simulink model "SF042A_HwAgSnsrls"  (R2013b)
settings: Solver=FixedStepDiscrete  SolverMode=SingleTasking  StartTime=0.0  StopTime=1  FixedStep=0.002  RelTol=1e-3
values from neighbouring files (symbols this model uses):
  ARCHGLBPRM_2MILLISEC_SEC_F32 = DataDict.Constant    [SF042A_HwAgSnsrls_DataDict.m]
  CORRDPINIONAGCON_CNT_U08 = DataDict.Constant    [SF042A_HwAgSnsrls_DataDict.m]
  FCENTROFFSCON_CNT_U08 = DataDict.Constant    [SF042A_HwAgSnsrls_DataDict.m]
  HwAgSnsrlsCorrdPinionAgHwConf = DataDict.Calibration    [SF042A_HwAgSnsrls_DataDict.m]
  HwAgSnsrlsFCentrHwConf = DataDict.Calibration    [SF042A_HwAgSnsrls_DataDict.m]
  HwAgSnsrlsSmotngCoeff = DataDict.Calibration    [SF042A_HwAgSnsrls_DataDict.m]
  HwAgSnsrlsSmotngStepThd = DataDict.Calibration    [SF042A_HwAgSnsrls_DataDict.m]
  HwAgSnsrlsStordPinionConf = DataDict.Calibration    [SF042A_HwAgSnsrls_DataDict.m]
  HwAgSnsrlsStordPinionConfThd = DataDict.Calibration    [SF042A_HwAgSnsrls_DataDict.m]
  HwAgSnsrlsVehDynDifThd = DataDict.Calibration    [SF042A_HwAgSnsrls_DataDict.m]
  HwAgSnsrlsVehDynHwConf = DataDict.Calibration    [SF042A_HwAgSnsrls_DataDict.m]
  HwAgSnsrlsVehDynMotVelThd = DataDict.Calibration    [SF042A_HwAgSnsrls_DataDict.m]
  HwAgSnsrlsVehDynPinionTqThd = DataDict.Calibration    [SF042A_HwAgSnsrls_DataDict.m]
  HwAgSnsrlsVehDynTmr1Thd = DataDict.Calibration    [SF042A_HwAgSnsrls_DataDict.m]
  HwAgSnsrlsVehDynTmr2Thd = DataDict.Calibration    [SF042A_HwAgSnsrls_DataDict.m]
  HwAgSnsrlsVehDynVehSpdThd = DataDict.Calibration    [SF042A_HwAgSnsrls_DataDict.m]
  HwAgSnsrlsVehDynYawRateThd = DataDict.Calibration    [SF042A_HwAgSnsrls_DataDict.m]
  HwAgSnsrlsWhlFrqThd = DataDict.Calibration    [SF042A_HwAgSnsrls_DataDict.m]
  HwAgSnsrlsWhlSpdHwAgCoeff1 = DataDict.Calibration    [SF042A_HwAgSnsrls_DataDict.m]
  HwAgSnsrlsWhlSpdHwAgCoeff2 = DataDict.Calibration    [SF042A_HwAgSnsrls_DataDict.m]
  HwAgSnsrlsWhlSpdHwAgThd = DataDict.Calibration    [SF042A_HwAgSnsrls_DataDict.m]
  HwAgSnsrlsWhlSpdHwConf = DataDict.Calibration    [SF042A_HwAgSnsrls_DataDict.m]
  HwAgSnsrlsWhlSpdRatThd = DataDict.Calibration    [SF042A_HwAgSnsrls_DataDict.m]
  HwAgSnsrlsWhlSpdTmrThd = DataDict.Calibration    [SF042A_HwAgSnsrls_DataDict.m]
  HwAgSnsrlsWhlSpdVehSpdThd = DataDict.Calibration    [SF042A_HwAgSnsrls_DataDict.m]
  LASTPOSNCON_CNT_U08 = DataDict.Constant    [SF042A_HwAgSnsrls_DataDict.m]
  MILLISECTO100MICROSEC_ULS_U32 = DataDict.Constant    [SF042A_HwAgSnsrls_DataDict.m]
  SysGlbPrmSysKineRat = DataDict.ImprtdCal    [SF042A_HwAgSnsrls_DataDict.m]
  SysGlbPrmSysTqRat = DataDict.ImprtdCal    [SF042A_HwAgSnsrls_DataDict.m]
  VEHDYNCON_CNT_U08 = DataDict.Constant    [SF042A_HwAgSnsrls_DataDict.m]
  WHLSPDCON_CNT_U08 = DataDict.Constant    [SF042A_HwAgSnsrls_DataDict.m]
undefined symbols (not defined in the file or in its folder): NtcNr1, SigQlfr1
libraries: NxtrAbslt x11, Fil x8, NxtrLim x4, simulink x3, NxtrNvM x1, FixdToFloat x1
(part 5 of 6)

== system SF042A_HwAgSnsrls/HwAgSnsrls/HwAgSnsrlsPer1/Arbitrator/NewHwAgConf/HwAgOffsSeln/WheelSpeed ==
  Action Port : ActionPort  ActionType=case
  CopyRight2 : Subsystem  Description=|  mask(Copyright Information){none=on}
      | Copyright info block.                                               
      |                                                                     
      | Place copyright information at the top of every subsystem in design.
      mask prompts: none "No parameters"
      mask help: Place copyright information at the top of every subsystem in design.
      mask Display:
      | NxtrConf = 'Nexteer Confidential';
      | 
      | sys = bdroot; %handle for the current model ("system")
      | first = get_param(sys,'Created');
      | if(isempty(first))
      |     first = datestr(now,'yyyy');
      | else
      |     first = first(end-3:end);  %year is last four digits
      | end
      | 
      | last = get_param(sys,'LastModifiedDate');
      | if isempty(last)
      |     last = datestr(now,'yyyy');
      | else
      |     last = last(end-3:end);
      | end
      | 
      | if strcmp(first,last)
      |     fprintf('%s -- Copyright %s Nexteer',NxtrConf,first)
      | else
      |     fprintf('%s -- %s%s- %s Nexteer',NxtrConf,char(169),first,last)
      | end
  Data Store Read1 : DataStoreRead  DataStoreName=WhlSpdHwAgOffs
  HwAgOffs : Outport
  wires:
  Data Store Read1/1 -> HwAgOffs/1

== system SF042A_HwAgSnsrls/HwAgSnsrls/HwAgSnsrlsPer1/RelHwAgCalcn/UseMotAg/GetMotAgOffs/CopyRight2 ==

== system SF042A_HwAgSnsrls/HwAgSnsrls/HwAgSnsrlsPer1/VehDynAutoCentr/LpFilOne/If Action Subsystem1/CopyRight2 ==

== system SF042A_HwAgSnsrls/HwAgSnsrls/HwAgSnsrlsPer1/VehDynAutoCentr/LpFilOne/If Action Subsystem2/CopyRight2 ==

== system SF042A_HwAgSnsrls/HwAgSnsrls/HwAgSnsrlsPer1/VehDynAutoCentr/LpFilOneEna/VehDynTmr1/CopyRight2 ==

== system SF042A_HwAgSnsrls/HwAgSnsrls/HwAgSnsrlsPer1/VehDynAutoCentr/LpFilOneEna/VehDynTmr1/GetTiSpan1 ==
  Action Port : ActionPort  ActionType=then
  CopyRight2 : Subsystem  Description=|  mask(Copyright Information){none=on}
      | Copyright info block.                                               
      |                                                                     
      | Place copyright information at the top of every subsystem in design.
      mask prompts: none "No parameters"
      mask help: Place copyright information at the top of every subsystem in design.
      mask Display:
      | NxtrConf = 'Nexteer Confidential';
      | 
      | sys = bdroot; %handle for the current model ("system")
      | first = get_param(sys,'Created');
      | if(isempty(first))
      |     first = datestr(now,'yyyy');
      | else
      |     first = first(end-3:end);  %year is last four digits
      | end
      | 
      | last = get_param(sys,'LastModifiedDate');
      | if isempty(last)
      |     last = datestr(now,'yyyy');
      | else
      |     last = last(end-3:end);
      | end
      | 
      | if strcmp(first,last)
      |     fprintf('%s -- Copyright %s Nexteer',NxtrConf,first)
      | else
      |     fprintf('%s -- %s%s- %s Nexteer',NxtrConf,char(169),first,last)
      | end
  Data Store Read : DataStoreRead  RequirementInfo={} %GIDa_74142626_ca52_4bba_8d6e_2554ddb3abed  DataStoreName=VehDynRefTmr1
  GetTiSpan100MicroSec32bit : Subsystem  RequirementInfo={} %GIDa_b1f833b8_7400_4722_b0de_2bfd26e0a16e  mask(Timer_GTS){}
      mask help: Used to get the time span between start and current time.
  Out1 : Outport
  wires:
  GetTiSpan100MicroSec32bit/1(TiSpan) -> Out1/1
  Data Store Read/1 -> GetTiSpan100MicroSec32bit/1(RefTmr)

== system SF042A_HwAgSnsrls/HwAgSnsrls/HwAgSnsrlsPer1/VehDynAutoCentr/LpFilOneEna/VehDynTmr1/If Action Subsystem3 ==
  RelHwAg : Inport
  Action Port : ActionPort  ActionType=then
  Constant1 : Constant  RequirementInfo="{'linktype_rmi_doors' '00012961 (/E-STEER Core/SubSystem Specifications/Application Functions - EA4/SF042A Handwheel Angle Sensorless)' '#SF042A_74' 'true' 'REQ:  SF042A_74' '' } %GIDa_bf3e4162_a852_43d6_8080_5a7c9c1c5760"  Value=false  OutDataTypeStr=boolean
      settings: AttributesFormatString=%<OutDataTypeStr>
  CopyRight2 : Subsystem  Description=|  mask(Copyright Information){none=on}
      | Copyright info block.                                               
      |                                                                     
      | Place copyright information at the top of every subsystem in design.
      mask prompts: none "No parameters"
      mask help: Place copyright information at the top of every subsystem in design.
      mask Display:
      | NxtrConf = 'Nexteer Confidential';
      | 
      | sys = bdroot; %handle for the current model ("system")
      | first = get_param(sys,'Created');
      | if(isempty(first))
      |     first = datestr(now,'yyyy');
      | else
      |     first = first(end-3:end);  %year is last four digits
      | end
      | 
      | last = get_param(sys,'LastModifiedDate');
      | if isempty(last)
      |     last = datestr(now,'yyyy');
      | else
      |     last = last(end-3:end);
      | end
      | 
      | if strcmp(first,last)
      |     fprintf('%s -- Copyright %s Nexteer',NxtrConf,first)
      | else
      |     fprintf('%s -- %s%s- %s Nexteer',NxtrConf,char(169),first,last)
      | end
  Data Store Write : DataStoreWrite  RequirementInfo="{'linktype_rmi_doors' '00012961 (/E-STEER Core/SubSystem Specifications/Application Functions - EA4/SF042A Handwheel Angle Sensorless)' '#SF042A_74' 'true' 'REQ:  SF042A_74' '' } %GIDa_355dd3a5_df19_4bc0_96c9_80662073f861"  DataStoreName=RelHwAgFil1  DataStoreElements=RelHwAgFil1.FilSt
  Data Store Write1 : DataStoreWrite  RequirementInfo="{'linktype_rmi_doors' '00012961 (/E-STEER Core/SubSystem Specifications/Application Functions - EA4/SF042A Handwheel Angle Sensorless)' '#SF042A_74' 'true' 'REQ:  SF042A_74' '' } %GIDa_2fc295c5_da8d_4166_ba51_0973e58fd4a2"  DataStoreName=VehDynRefTmr2
  Data Store Write2 : DataStoreWrite  RequirementInfo="{'linktype_rmi_doors' '00012961 (/E-STEER Core/SubSystem Specifications/Application Functions - EA4/SF042A Handwheel Angle Sensorless)' '#SF042A_74' 'true' 'REQ:  SF042A_74' '' } %GIDa_f80ae885_8ebf_478b_9b31_2b213f41a136"  DataStoreName=PrevVehDynFil1Ena
  GetRefTmr100MicroSec32bit : Subsystem  RequirementInfo="{'linktype_rmi_doors' '00012961 (/E-STEER Core/SubSystem Specifications/Application Functions - EA4/SF042A Handwheel Angle Sensorless)' '#SF042A_74' 'true' 'REQ:  SF042A_74' '' } %GIDa_22af453f_e23e_4d39_aa78_6aee3b18adc7"  mask(Timer_GRF){}
      mask help: Used to get the reference time in a model.
  wires:
  Constant1/1 -> Data Store Write2/1
  GetRefTmr100MicroSec32bit/1(RefTmr) -> Data Store Write1/1
  RelHwAg/1 -> Data Store Write/1

== system SF042A_HwAgSnsrls/HwAgSnsrls/HwAgSnsrlsPer1/VehDynAutoCentr/LpFilOneEna/VehDynTmr1/Set to 0 ==
  Action Port : ActionPort  ActionType=else
  Constant= : Constant  RequirementInfo={} %GIDa_d225d475_710f_4e18_8d33_cdb597cd94b8  Value=0  OutDataTypeStr=uint32
      settings: AttributesFormatString=%<OutDataTypeStr>
  CopyRight2 : Subsystem  Description=|  mask(Copyright Information){none=on}
      | Copyright info block.                                               
      |                                                                     
      | Place copyright information at the top of every subsystem in design.
      mask prompts: none "No parameters"
      mask help: Place copyright information at the top of every subsystem in design.
      mask Display:
      | NxtrConf = 'Nexteer Confidential';
      | 
      | sys = bdroot; %handle for the current model ("system")
      | first = get_param(sys,'Created');
      | if(isempty(first))
      |     first = datestr(now,'yyyy');
      | else
      |     first = first(end-3:end);  %year is last four digits
      | end
      | 
      | last = get_param(sys,'LastModifiedDate');
      | if isempty(last)
      |     last = datestr(now,'yyyy');
      | else
      |     last = last(end-3:end);
      | end
      | 
      | if strcmp(first,last)
      |     fprintf('%s -- Copyright %s Nexteer',NxtrConf,first)
      | else
      |     fprintf('%s -- %s%s- %s Nexteer',NxtrConf,char(169),first,last)
      | end
  Data Store Write1 : DataStoreWrite  RequirementInfo={} %GIDa_09f33c30_f3bd_43b6_b205_fca292d21401  DataStoreName=VehDynRefTmr1
  GetRefTmr100MicroSec32bit : Subsystem  RequirementInfo={} %GIDa_a927190b_d792_495c_8b1d_712b059613e1  mask(Timer_GRF){}
      mask help: Used to get the reference time in a model.
  Out1 : Outport
  wires:
  GetRefTmr100MicroSec32bit/1(RefTmr) -> Data Store Write1/1
  Constant=/1 -> Out1/1

== system SF042A_HwAgSnsrls/HwAgSnsrls/HwAgSnsrlsPer1/VehDynAutoCentr/LpFilTwo/If Action Subsystem3/CopyRight2 ==

== system SF042A_HwAgSnsrls/HwAgSnsrls/HwAgSnsrlsPer1/VehDynAutoCentr/LpFilTwo/If Action Subsystem4/CopyRight2 ==

== system SF042A_HwAgSnsrls/HwAgSnsrls/HwAgSnsrlsPer1/VehDynAutoCentr/LpFilTwoEna/VehDynTmr2/CopyRight2 ==

== system SF042A_HwAgSnsrls/HwAgSnsrls/HwAgSnsrlsPer1/VehDynAutoCentr/LpFilTwoEna/VehDynTmr2/GetTiSpan2 ==
  Action Port : ActionPort  ActionType=then
  CopyRight2 : Subsystem  Description=|  mask(Copyright Information){none=on}
      | Copyright info block.                                               
      |                                                                     
      | Place copyright information at the top of every subsystem in design.
      mask prompts: none "No parameters"
      mask help: Place copyright information at the top of every subsystem in design.
      mask Display:
      | NxtrConf = 'Nexteer Confidential';
      | 
      | sys = bdroot; %handle for the current model ("system")
      | first = get_param(sys,'Created');
      | if(isempty(first))
      |     first = datestr(now,'yyyy');
      | else
      |     first = first(end-3:end);  %year is last four digits
      | end
      | 
      | last = get_param(sys,'LastModifiedDate');
      | if isempty(last)
      |     last = datestr(now,'yyyy');
      | else
      |     last = last(end-3:end);
      | end
      | 
      | if strcmp(first,last)
      |     fprintf('%s -- Copyright %s Nexteer',NxtrConf,first)
      | else
      |     fprintf('%s -- %s%s- %s Nexteer',NxtrConf,char(169),first,last)
      | end
  Data Store Read : DataStoreRead  DataStoreName=VehDynRefTmr2
  GetTiSpan100MicroSec32bit : Subsystem  mask(Timer_GTS){}
      mask help: Used to get the time span between start and current time.
  Out1 : Outport
  wires:
  GetTiSpan100MicroSec32bit/1(TiSpan) -> Out1/1
  Data Store Read/1 -> GetTiSpan100MicroSec32bit/1(RefTmr)

== system SF042A_HwAgSnsrls/HwAgSnsrls/HwAgSnsrlsPer1/VehDynAutoCentr/LpFilTwoEna/VehDynTmr2/If Action Subsystem4 ==
  FildRelHwAg1 : Inport
  Action Port : ActionPort  ActionType=then
  Constant1 : Constant  Value=false  OutDataTypeStr=boolean
      settings: AttributesFormatString=%<OutDataTypeStr>
  CopyRight2 : Subsystem  Description=|  mask(Copyright Information){none=on}
      | Copyright info block.                                               
      |                                                                     
      | Place copyright information at the top of every subsystem in design.
      mask prompts: none "No parameters"
      mask help: Place copyright information at the top of every subsystem in design.
      mask Display:
      | NxtrConf = 'Nexteer Confidential';
      | 
      | sys = bdroot; %handle for the current model ("system")
      | first = get_param(sys,'Created');
      | if(isempty(first))
      |     first = datestr(now,'yyyy');
      | else
      |     first = first(end-3:end);  %year is last four digits
      | end
      | 
      | last = get_param(sys,'LastModifiedDate');
      | if isempty(last)
      |     last = datestr(now,'yyyy');
      | else
      |     last = last(end-3:end);
      | end
      | 
      | if strcmp(first,last)
      |     fprintf('%s -- Copyright %s Nexteer',NxtrConf,first)
      | else
      |     fprintf('%s -- %s%s- %s Nexteer',NxtrConf,char(169),first,last)
      | end
  Data Store Write : DataStoreWrite  DataStoreName=RelHwAgFil2  DataStoreElements=RelHwAgFil2.FilSt
  Data Store Write1 : DataStoreWrite  DataStoreName=PrevVehDynFil2Ena
  wires:
  Constant1/1 -> Data Store Write1/1
  FildRelHwAg1/1 -> Data Store Write/1

== system SF042A_HwAgSnsrls/HwAgSnsrls/HwAgSnsrlsPer1/VehDynAutoCentr/LpFilTwoEna/VehDynTmr2/Set to 0 ==
  Action Port : ActionPort  ActionType=else
  Constant= : Constant  Value=0  OutDataTypeStr=uint32
      settings: AttributesFormatString=%<OutDataTypeStr>
  CopyRight2 : Subsystem  Description=|  mask(Copyright Information){none=on}
      | Copyright info block.                                               
      |                                                                     
      | Place copyright information at the top of every subsystem in design.
      mask prompts: none "No parameters"
      mask help: Place copyright information at the top of every subsystem in design.
      mask Display:
      | NxtrConf = 'Nexteer Confidential';
      | 
      | sys = bdroot; %handle for the current model ("system")
      | first = get_param(sys,'Created');
      | if(isempty(first))
      |     first = datestr(now,'yyyy');
      | else
      |     first = first(end-3:end);  %year is last four digits
      | end
      | 
      | last = get_param(sys,'LastModifiedDate');
      | if isempty(last)
      |     last = datestr(now,'yyyy');
      | else
      |     last = last(end-3:end);
      | end
      | 
      | if strcmp(first,last)
      |     fprintf('%s -- Copyright %s Nexteer',NxtrConf,first)
      | else
      |     fprintf('%s -- %s%s- %s Nexteer',NxtrConf,char(169),first,last)
      | end
  Data Store Write1 : DataStoreWrite  DataStoreName=VehDynRefTmr2
  GetRefTmr100MicroSec32bit : Subsystem  mask(Timer_GRF){}
      mask help: Used to get the reference time in a model.
  Out1 : Outport
  wires:
  GetRefTmr100MicroSec32bit/1(RefTmr) -> Data Store Write1/1
  Constant=/1 -> Out1/1

== system SF042A_HwAgSnsrls/HwAgSnsrls/HwAgSnsrlsPer1/WhlSpdAutoCentr/WhlSpd/If Action Subsystem/CopyRight2 ==

== system SF042A_HwAgSnsrls/HwAgSnsrls/HwAgSnsrlsPer1/WhlSpdAutoCentr/WhlSpd/If Action Subsystem1/CopyRight2 ==

== system SF042A_HwAgSnsrls/HwAgSnsrls/HwAgSnsrlsPer1/WhlSpdAutoCentr/WhlSpd/If Action Subsystem1/If Action Subsystem3 ==
  WhlSpdCalcdHwAg : Inport  RequirementInfo={'linktype_rmi_doors' '00012961 (/E-STEER Core/SubSystem Specifications/Application Functions - EA4/SF042A Handwheel Angle Sensorless)' '#SF042A_70' 'true' 'REQ: SF042A_70' '' } %GIDa_7cd06f39_2218_4fea_b136_f484ec17fff2
  RelHwAg : Inport  RequirementInfo={'linktype_rmi_doors' '00012961 (/E-STEER Core/SubSystem Specifications/Application Functions - EA4/SF042A Handwheel Angle Sensorless)' '#SF042A_70' 'true' 'REQ: SF042A_70' '' } %GIDa_cc8e37a6_8bbd_4338_bf0c_7d37568d3593  Port=2
  Action Port : ActionPort  ActionType=then
  Add1 : Sum  RequirementInfo={'linktype_rmi_doors' '00012961 (/E-STEER Core/SubSystem Specifications/Application Functions - EA4/SF042A Handwheel Angle Sensorless)' '#SF042A_70' 'true' 'REQ: SF042A_70' '' } %GIDa_3841f18f_86ea_4899_addd_b0841663b9d4  Inputs=+-
  Constant1 : Constant  RequirementInfo={'linktype_rmi_doors' '00012961 (/E-STEER Core/SubSystem Specifications/Application Functions - EA4/SF042A Handwheel Angle Sensorless)' '#SF042A_70' 'true' 'REQ: SF042A_70' '' } %GIDa_14d4ec9e_5312_4daf_aca9_bd2a7bb746ee  Value=HwAgSnsrlsWhlSpdHwConf
  Constant2 : Constant  RequirementInfo={'linktype_rmi_doors' '00012961 (/E-STEER Core/SubSystem Specifications/Application Functions - EA4/SF042A Handwheel Angle Sensorless)' '#SF042A_70' 'true' 'REQ: SF042A_70' '' } %GIDa_fd363aae_15e5_4022_9e3e_50f897442608  Value=false  OutDataTypeStr=boolean
      settings: AttributesFormatString=%<OutDataTypeStr>
  CopyRight2 : Subsystem  Description=|  mask(Copyright Information){none=on}
      | Copyright info block.                                               
      |                                                                     
      | Place copyright information at the top of every subsystem in design.
      mask prompts: none "No parameters"
      mask help: Place copyright information at the top of every subsystem in design.
      mask Display:
      | NxtrConf = 'Nexteer Confidential';
      | 
      | sys = bdroot; %handle for the current model ("system")
      | first = get_param(sys,'Created');
      | if(isempty(first))
      |     first = datestr(now,'yyyy');
      | else
      |     first = first(end-3:end);  %year is last four digits
      | end
      | 
      | last = get_param(sys,'LastModifiedDate');
      | if isempty(last)
      |     last = datestr(now,'yyyy');
      | else
      |     last = last(end-3:end);
      | end
      | 
      | if strcmp(first,last)
      |     fprintf('%s -- Copyright %s Nexteer',NxtrConf,first)
      | else
      |     fprintf('%s -- %s%s- %s Nexteer',NxtrConf,char(169),first,last)
      | end
  Data Store Write : DataStoreWrite  RequirementInfo={'linktype_rmi_doors' '00012961 (/E-STEER Core/SubSystem Specifications/Application Functions - EA4/SF042A Handwheel Angle Sensorless)' '#SF042A_70' 'true' 'REQ: SF042A_70' '' } %GIDa_a6677650_af95_4501_b8c3_0c54457055f9  DataStoreName=WhlSpdHwAgOffs
  Data Store Write1 : DataStoreWrite  RequirementInfo={'linktype_rmi_doors' '00012961 (/E-STEER Core/SubSystem Specifications/Application Functions - EA4/SF042A Handwheel Angle Sensorless)' '#SF042A_70' 'true' 'REQ: SF042A_70' '' } %GIDa_3a32dbe7_0549_46a1_8f4c_ed050cc79bfd  DataStoreName=WhlSpdHwAgLrndEna
  Data Store Write2 : DataStoreWrite  RequirementInfo={'linktype_rmi_doors' '00012961 (/E-STEER Core/SubSystem Specifications/Application Functions - EA4/SF042A Handwheel Angle Sensorless)' '#SF042A_70' 'true' 'REQ: SF042A_70' '' } %GIDa_af951123_ddd0_4dbe_9eec_6118f409597e  DataStoreName=WhlSpdHwConf
  wires:
  Constant1/1 -> Data Store Write2/1
  Add1/1 -> Data Store Write/1
  WhlSpdCalcdHwAg/1 -> Add1/2
  RelHwAg/1 -> Add1/1
  Constant2/1 -> Data Store Write1/1

== system SF042A_HwAgSnsrls/HwAgSnsrls/HwAgSnsrlsPer1/WhlSpdAutoCentr/WhlSpd/Output 0/CopyRight2 ==

== system SF042A_HwAgSnsrls/HwAgSnsrls/HwAgSnsrlsPer1/WhlSpdAutoCentr/WhlSpd/VehSpdChk/CopyRight2 ==

== system SF042A_HwAgSnsrls/HwAgSnsrls/HwAgSnsrlsPer1/WhlSpdAutoCentr/WhlSpd/VehSpdChk/GetTiSpan  ==
  Action Port : ActionPort  ActionType=then
  CopyRight2 : Subsystem  Description=|  mask(Copyright Information){none=on}
      | Copyright info block.                                               
      |                                                                     
      | Place copyright information at the top of every subsystem in design.
      mask prompts: none "No parameters"
      mask help: Place copyright information at the top of every subsystem in design.
      mask Display:
      | NxtrConf = 'Nexteer Confidential';
      | 
      | sys = bdroot; %handle for the current model ("system")
      | first = get_param(sys,'Created');
      | if(isempty(first))
      |     first = datestr(now,'yyyy');
      | else
      |     first = first(end-3:end);  %year is last four digits
      | end
      | 
      | last = get_param(sys,'LastModifiedDate');
      | if isempty(last)
      |     last = datestr(now,'yyyy');
      | else
      |     last = last(end-3:end);
      | end
      | 
      | if strcmp(first,last)
      |     fprintf('%s -- Copyright %s Nexteer',NxtrConf,first)
      | else
      |     fprintf('%s -- %s%s- %s Nexteer',NxtrConf,char(169),first,last)
      | end
  Data Store Read : DataStoreRead  RequirementInfo={'linktype_rmi_doors' '00012961 (/E-STEER Core/SubSystem Specifications/Application Functions - EA4/SF042A Handwheel Angle Sensorless)' '#SF042A_70' 'true' 'REQ: SF042A_70' '' } %GIDa_3ca63f87_39e3_409a_9160_18ba87e890c0  DataStoreName=WhlSpdRefTmr
  GetTiSpan100MicroSec32bit : Subsystem  RequirementInfo={'linktype_rmi_doors' '00012961 (/E-STEER Core/SubSystem Specifications/Application Functions - EA4/SF042A Handwheel Angle Sensorless)' '#SF042A_70' 'true' 'REQ: SF042A_70' '' } %GIDa_edd8e882_0a03_4e06_a52f_74ba6a298fda  mask(Timer_GTS){}
      mask help: Used to get the time span between start and current time.
  Out1 : Outport  RequirementInfo={'linktype_rmi_doors' '00012961 (/E-STEER Core/SubSystem Specifications/Application Functions - EA4/SF042A Handwheel Angle Sensorless)' '#SF042A_70' 'true' 'REQ: SF042A_70' '' } %GIDa_e3898572_f33b_41bc_8d76_8d60318fc428
  wires:
  Data Store Read/1 -> GetTiSpan100MicroSec32bit/1(RefTmr)
  GetTiSpan100MicroSec32bit/1(TiSpan) -> Out1/1

== system SF042A_HwAgSnsrls/HwAgSnsrls/HwAgSnsrlsPer1/WhlSpdAutoCentr/WhlSpd/VehSpdChk/Set to 0 ==
  Action Port : ActionPort  ActionType=else
  Constant : Constant  RequirementInfo={'linktype_rmi_doors' '00012961 (/E-STEER Core/SubSystem Specifications/Application Functions - EA4/SF042A Handwheel Angle Sensorless)' '#SF042A_70' 'true' 'REQ: SF042A_70' '' } %GIDa_d2d8b80d_a37a_4d9c_85b2_1be7d46366e3  Value=0  OutDataTypeStr=uint32
      settings: AttributesFormatString=%<OutDataTypeStr>
  CopyRight2 : Subsystem  Description=|  mask(Copyright Information){none=on}
      | Copyright info block.                                               
      |                                                                     
      | Place copyright information at the top of every subsystem in design.
      mask prompts: none "No parameters"
      mask help: Place copyright information at the top of every subsystem in design.
      mask Display:
      | NxtrConf = 'Nexteer Confidential';
      | 
      | sys = bdroot; %handle for the current model ("system")
      | first = get_param(sys,'Created');
      | if(isempty(first))
      |     first = datestr(now,'yyyy');
      | else
      |     first = first(end-3:end);  %year is last four digits
      | end
      | 
      | last = get_param(sys,'LastModifiedDate');
      | if isempty(last)
      |     last = datestr(now,'yyyy');
      | else
      |     last = last(end-3:end);
      | end
      | 
      | if strcmp(first,last)
      |     fprintf('%s -- Copyright %s Nexteer',NxtrConf,first)
      | else
      |     fprintf('%s -- %s%s- %s Nexteer',NxtrConf,char(169),first,last)
      | end
  Data Store Write : DataStoreWrite  RequirementInfo={'linktype_rmi_doors' '00012961 (/E-STEER Core/SubSystem Specifications/Application Functions - EA4/SF042A Handwheel Angle Sensorless)' '#SF042A_70' 'true' 'REQ: SF042A_70' '' } %GIDa_bc610a1d_c533_4119_9c55_dd67f6777192  DataStoreName=WhlSpdRefTmr
  GetRefTmr100MicroSec32bit : Subsystem  RequirementInfo={'linktype_rmi_doors' '00012961 (/E-STEER Core/SubSystem Specifications/Application Functions - EA4/SF042A Handwheel Angle Sensorless)' '#SF042A_70' 'true' 'REQ: SF042A_70' '' } %GIDa_7ddd2f5b_e599_4714_b3cd_a7c77aa813ff  mask(Timer_GRF){}
      mask help: Used to get the reference time in a model.
  Out1 : Outport  RequirementInfo={'linktype_rmi_doors' '00012961 (/E-STEER Core/SubSystem Specifications/Application Functions - EA4/SF042A Handwheel Angle Sensorless)' '#SF042A_70' 'true' 'REQ: SF042A_70' '' } %GIDa_d8f1dd78_590f_497f_9773_2aa306803993
  wires:
  GetRefTmr100MicroSec32bit/1(RefTmr) -> Data Store Write/1
  Constant/1 -> Out1/1

== system SF042A_HwAgSnsrls/HwAgSnsrls/HwAgSnsrlsPer1/Arbitrator/NewHwAgConf/HwAgOffsSeln/CorrectedPinionAg/CopyRight2 ==

== system SF042A_HwAgSnsrls/HwAgSnsrls/HwAgSnsrlsPer1/Arbitrator/NewHwAgConf/HwAgOffsSeln/ForcedCenter/CopyRight2 ==

== system SF042A_HwAgSnsrls/HwAgSnsrls/HwAgSnsrlsPer1/Arbitrator/NewHwAgConf/HwAgOffsSeln/StordLastPosn/CopyRight2 ==

== system SF042A_HwAgSnsrls/HwAgSnsrls/HwAgSnsrlsPer1/Arbitrator/NewHwAgConf/HwAgOffsSeln/VehicleDynamic/CopyRight2 ==

== system SF042A_HwAgSnsrls/HwAgSnsrls/HwAgSnsrlsPer1/Arbitrator/NewHwAgConf/HwAgOffsSeln/WheelSpeed/CopyRight2 ==

== system SF042A_HwAgSnsrls/HwAgSnsrls/HwAgSnsrlsPer1/VehDynAutoCentr/LpFilOneEna/VehDynTmr1/GetTiSpan1/CopyRight2 ==

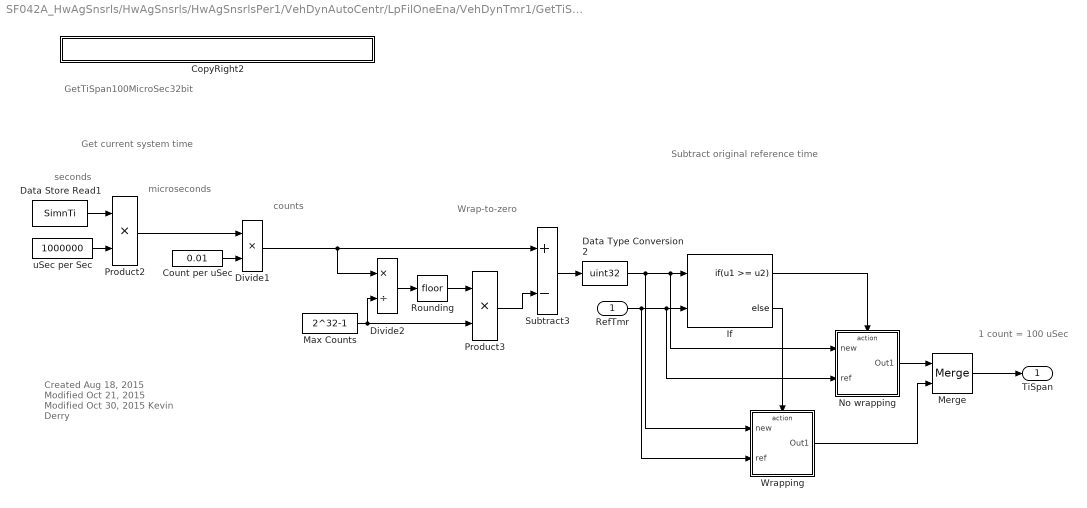
== system SF042A_HwAgSnsrls/HwAgSnsrls/HwAgSnsrlsPer1/VehDynAutoCentr/LpFilOneEna/VehDynTmr1/GetTiSpan1/GetTiSpan100MicroSec32bit ==
  note: Subtract original reference time
  note: seconds
  note: microseconds
  note: counts
  note: Wrap-to-zero
  note: 1 count = 100 uSec
  note: Get current system time
  note: GetTiSpan100MicroSec32bit
  note: Created Aug 18, 2015
      | Modified Oct 21, 2015
      | Modified Oct 30, 2015
      | Kevin Derry
  RefTmr : Inport
  CopyRight2 : Subsystem  Description=|  mask(Copyright Information){none=on}
      | Copyright info block.                                               
      |                                                                     
      | Place copyright information at the top of every subsystem in design.
      mask prompts: none "No parameters"
      mask help: Place copyright information at the top of every subsystem in design.
      mask Display:
      | NxtrConf = 'Nexteer Confidential';
      | 
      | sys = bdroot; %handle for the current model ("system")
      | first = get_param(sys,'Created');
      | if(isempty(first))
      |     first = datestr(now,'yyyy');
      | else
      |     first = first(end-3:end);  %year is last four digits
      | end
      | 
      | last = get_param(sys,'LastModifiedDate');
      | if isempty(last)
      |     last = datestr(now,'yyyy');
      | else
      |     last = last(end-3:end);
      | end
      | 
      | if strcmp(first,last)
      |     fprintf('%s -- Copyright %s Nexteer',NxtrConf,first)
      | else
      |     fprintf('%s -- %s%s- %s Nexteer',NxtrConf,char(169),first,last)
      | end
  Count per uSec : Constant  Value=0.01
  Data Store Read1 : DataStoreRead  DataStoreName=SimnTi
  Data Type Conversion2 : DataTypeConversion  OutDataTypeStr=uint32
  Divide1 : Product  Inputs=**
  Divide2 : Product  Inputs=*/
  If : If  NumInputs=2  IfExpression=u1 >= u2
  Max Counts : Constant  Value=2^32-1
  Merge : Merge
  No wrapping : Subsystem  TreatAsAtomicUnit=on
  Product2 : Product
  Product3 : Product
  Rounding : Rounding
  Subtract3 : Sum  Inputs=+-
  Wrapping : Subsystem  TreatAsAtomicUnit=on
  uSec per Sec : Constant  Value=1000000
  TiSpan : Outport
  wires:
  Wrapping/1(Out1) -> Merge/2
  No wrapping/1(Out1) -> Merge/1
  If/2 -> Wrapping/Action
  If/1 -> No wrapping/Action
  Product3/1 -> Subtract3/2
  Subtract3/1 -> Data Type Conversion2/1
  Rounding/1 -> Product3/1
  Divide2/1 -> Rounding/1
  Max Counts/1 -> Divide2/2, Product3/2
  Divide1/1 -> Divide2/1, Subtract3/1
  Product2/1 -> Divide1/1
  Data Store Read1/1 -> Product2/1
  Count per uSec/1 -> Divide1/2
  uSec per Sec/1 -> Product2/2
  Merge/1 -> TiSpan/1
  RefTmr/1 -> If/2, No wrapping/2(ref), Wrapping/2(ref)
  Data Type Conversion2/1 -> If/1, No wrapping/1(new), Wrapping/1(new)

== system SF042A_HwAgSnsrls/HwAgSnsrls/HwAgSnsrlsPer1/VehDynAutoCentr/LpFilOneEna/VehDynTmr1/If Action Subsystem3/CopyRight2 ==

== system SF042A_HwAgSnsrls/HwAgSnsrls/HwAgSnsrlsPer1/VehDynAutoCentr/LpFilOneEna/VehDynTmr1/If Action Subsystem3/GetRefTmr100MicroSec32bit ==
  note: 1 count = 100 uSec
  note: seconds
  note: microseconds
  note: counts
  note: Wrap-to-zero
  note: GetRefTmr100MicroSec32bit
  note: Created Aug 18, 2015
      | Modified Oct 21, 2015
      | Modified Oct 30, 2015
      | Kevin Derry
  CopyRight2 : Subsystem  Description=|  mask(Copyright Information){none=on}
      | Copyright info block.                                               
      |                                                                     
      | Place copyright information at the top of every subsystem in design.
      mask prompts: none "No parameters"
      mask help: Place copyright information at the top of every subsystem in design.
      mask Display:
      | NxtrConf = 'Nexteer Confidential';
      | 
      | sys = bdroot; %handle for the current model ("system")
      | first = get_param(sys,'Created');
      | if(isempty(first))
      |     first = datestr(now,'yyyy');
      | else
      |     first = first(end-3:end);  %year is last four digits
      | end
      | 
      | last = get_param(sys,'LastModifiedDate');
      | if isempty(last)
      |     last = datestr(now,'yyyy');
      | else
      |     last = last(end-3:end);
      | end
      | 
      | if strcmp(first,last)
      |     fprintf('%s -- Copyright %s Nexteer',NxtrConf,first)
      | else
      |     fprintf('%s -- %s%s- %s Nexteer',NxtrConf,char(169),first,last)
      | end
  Count per uSec : Constant  Value=0.01
  Data Store Read1 : DataStoreRead  DataStoreName=SimnTi
  Data Type Conversion1 : DataTypeConversion  OutDataTypeStr=uint32
  Divide1 : Product  Inputs=**
  Divide2 : Product  Inputs=*/
  Max Counts : Constant  Value=2^32-1
  Product1 : Product
  Product2 : Product
  Rounding : Rounding
  Subtract1 : Sum  Inputs=+-
  uSec per Sec : Constant  Value=1000000
  RefTmr : Outport
  wires:
  Product2/1 -> Subtract1/2
  Subtract1/1 -> Data Type Conversion1/1
  Rounding/1 -> Product2/1
  Divide2/1 -> Rounding/1
  Max Counts/1 -> Divide2/2, Product2/2
  Divide1/1 -> Divide2/1, Subtract1/1
  Product1/1 -> Divide1/1
  Count per uSec/1 -> Divide1/2
  uSec per Sec/1 -> Product1/2
  Data Type Conversion1/1 -> RefTmr/1
  Data Store Read1/1 -> Product1/1

== system SF042A_HwAgSnsrls/HwAgSnsrls/HwAgSnsrlsPer1/VehDynAutoCentr/LpFilOneEna/VehDynTmr1/Set to 0/CopyRight2 ==

== system SF042A_HwAgSnsrls/HwAgSnsrls/HwAgSnsrlsPer1/VehDynAutoCentr/LpFilOneEna/VehDynTmr1/Set to 0/GetRefTmr100MicroSec32bit ==
  note: 1 count = 100 uSec
  note: seconds
  note: microseconds
  note: counts
  note: Wrap-to-zero
  note: GetRefTmr100MicroSec32bit
  note: Created Aug 18, 2015
      | Modified Oct 21, 2015
      | Modified Oct 30, 2015
      | Kevin Derry
  CopyRight2 : Subsystem  Description=|  mask(Copyright Information){none=on}
      | Copyright info block.                                               
      |                                                                     
      | Place copyright information at the top of every subsystem in design.
      mask prompts: none "No parameters"
      mask help: Place copyright information at the top of every subsystem in design.
      mask Display:
      | NxtrConf = 'Nexteer Confidential';
      | 
      | sys = bdroot; %handle for the current model ("system")
      | first = get_param(sys,'Created');
      | if(isempty(first))
      |     first = datestr(now,'yyyy');
      | else
      |     first = first(end-3:end);  %year is last four digits
      | end
      | 
      | last = get_param(sys,'LastModifiedDate');
      | if isempty(last)
      |     last = datestr(now,'yyyy');
      | else
      |     last = last(end-3:end);
      | end
      | 
      | if strcmp(first,last)
      |     fprintf('%s -- Copyright %s Nexteer',NxtrConf,first)
      | else
      |     fprintf('%s -- %s%s- %s Nexteer',NxtrConf,char(169),first,last)
      | end
  Count per uSec : Constant  Value=0.01
  Data Store Read1 : DataStoreRead  DataStoreName=SimnTi
  Data Type Conversion1 : DataTypeConversion  OutDataTypeStr=uint32
  Divide1 : Product  Inputs=**
  Divide2 : Product  Inputs=*/
  Max Counts : Constant  Value=2^32-1
  Product1 : Product
  Product2 : Product
  Rounding : Rounding
  Subtract1 : Sum  Inputs=+-
  uSec per Sec : Constant  Value=1000000
  RefTmr : Outport
  wires:
  Product2/1 -> Subtract1/2
  Subtract1/1 -> Data Type Conversion1/1
  Rounding/1 -> Product2/1
  Divide2/1 -> Rounding/1
  Max Counts/1 -> Divide2/2, Product2/2
  Divide1/1 -> Divide2/1, Subtract1/1
  Product1/1 -> Divide1/1
  Count per uSec/1 -> Divide1/2
  uSec per Sec/1 -> Product1/2
  Data Type Conversion1/1 -> RefTmr/1
  Data Store Read1/1 -> Product1/1

== system SF042A_HwAgSnsrls/HwAgSnsrls/HwAgSnsrlsPer1/VehDynAutoCentr/LpFilTwoEna/VehDynTmr2/GetTiSpan2/CopyRight2 ==

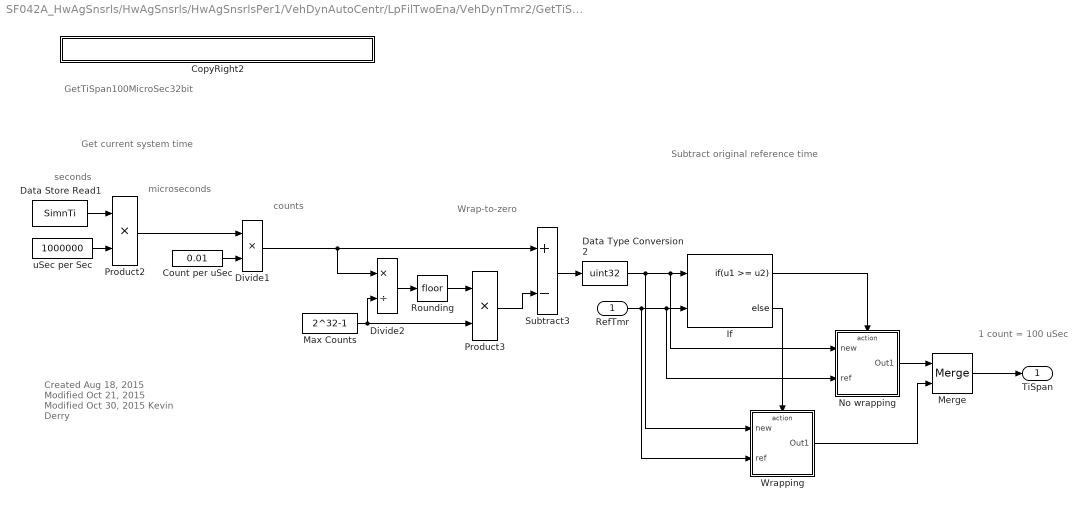
== system SF042A_HwAgSnsrls/HwAgSnsrls/HwAgSnsrlsPer1/VehDynAutoCentr/LpFilTwoEna/VehDynTmr2/GetTiSpan2/GetTiSpan100MicroSec32bit ==
  note: Subtract original reference time
  note: seconds
  note: microseconds
  note: counts
  note: Wrap-to-zero
  note: 1 count = 100 uSec
  note: Get current system time
  note: GetTiSpan100MicroSec32bit
  note: Created Aug 18, 2015
      | Modified Oct 21, 2015
      | Modified Oct 30, 2015
      | Kevin Derry
  RefTmr : Inport
  CopyRight2 : Subsystem  Description=|  mask(Copyright Information){none=on}
      | Copyright info block.                                               
      |                                                                     
      | Place copyright information at the top of every subsystem in design.
      mask prompts: none "No parameters"
      mask help: Place copyright information at the top of every subsystem in design.
      mask Display:
      | NxtrConf = 'Nexteer Confidential';
      | 
      | sys = bdroot; %handle for the current model ("system")
      | first = get_param(sys,'Created');
      | if(isempty(first))
      |     first = datestr(now,'yyyy');
      | else
      |     first = first(end-3:end);  %year is last four digits
      | end
      | 
      | last = get_param(sys,'LastModifiedDate');
      | if isempty(last)
      |     last = datestr(now,'yyyy');
      | else
      |     last = last(end-3:end);
      | end
      | 
      | if strcmp(first,last)
      |     fprintf('%s -- Copyright %s Nexteer',NxtrConf,first)
      | else
      |     fprintf('%s -- %s%s- %s Nexteer',NxtrConf,char(169),first,last)
      | end
  Count per uSec : Constant  Value=0.01
  Data Store Read1 : DataStoreRead  DataStoreName=SimnTi
  Data Type Conversion2 : DataTypeConversion  OutDataTypeStr=uint32
  Divide1 : Product  Inputs=**
  Divide2 : Product  Inputs=*/
  If : If  NumInputs=2  IfExpression=u1 >= u2
  Max Counts : Constant  Value=2^32-1
  Merge : Merge
  No wrapping : Subsystem  TreatAsAtomicUnit=on
  Product2 : Product
  Product3 : Product
  Rounding : Rounding
  Subtract3 : Sum  Inputs=+-
  Wrapping : Subsystem  TreatAsAtomicUnit=on
  uSec per Sec : Constant  Value=1000000
  TiSpan : Outport
  wires:
  Wrapping/1(Out1) -> Merge/2
  No wrapping/1(Out1) -> Merge/1
  If/2 -> Wrapping/Action
  If/1 -> No wrapping/Action
  Product3/1 -> Subtract3/2
  Subtract3/1 -> Data Type Conversion2/1
  Rounding/1 -> Product3/1
  Divide2/1 -> Rounding/1
  Max Counts/1 -> Divide2/2, Product3/2
  Divide1/1 -> Divide2/1, Subtract3/1
  Product2/1 -> Divide1/1
  Data Store Read1/1 -> Product2/1
  Count per uSec/1 -> Divide1/2
  uSec per Sec/1 -> Product2/2
  Merge/1 -> TiSpan/1
  RefTmr/1 -> If/2, No wrapping/2(ref), Wrapping/2(ref)
  Data Type Conversion2/1 -> If/1, No wrapping/1(new), Wrapping/1(new)

== system SF042A_HwAgSnsrls/HwAgSnsrls/HwAgSnsrlsPer1/VehDynAutoCentr/LpFilTwoEna/VehDynTmr2/If Action Subsystem4/CopyRight2 ==

== system SF042A_HwAgSnsrls/HwAgSnsrls/HwAgSnsrlsPer1/VehDynAutoCentr/LpFilTwoEna/VehDynTmr2/Set to 0/CopyRight2 ==

== system SF042A_HwAgSnsrls/HwAgSnsrls/HwAgSnsrlsPer1/VehDynAutoCentr/LpFilTwoEna/VehDynTmr2/Set to 0/GetRefTmr100MicroSec32bit ==
  note: 1 count = 100 uSec
  note: seconds
  note: microseconds
  note: counts
  note: Wrap-to-zero
  note: GetRefTmr100MicroSec32bit
  note: Created Aug 18, 2015
      | Modified Oct 21, 2015
      | Modified Oct 30, 2015
      | Kevin Derry
  CopyRight2 : Subsystem  Description=|  mask(Copyright Information){none=on}
      | Copyright info block.                                               
      |                                                                     
      | Place copyright information at the top of every subsystem in design.
      mask prompts: none "No parameters"
      mask help: Place copyright information at the top of every subsystem in design.
      mask Display:
      | NxtrConf = 'Nexteer Confidential';
      | 
      | sys = bdroot; %handle for the current model ("system")
      | first = get_param(sys,'Created');
      | if(isempty(first))
      |     first = datestr(now,'yyyy');
      | else
      |     first = first(end-3:end);  %year is last four digits
      | end
      | 
      | last = get_param(sys,'LastModifiedDate');
      | if isempty(last)
      |     last = datestr(now,'yyyy');
      | else
      |     last = last(end-3:end);
      | end
      | 
      | if strcmp(first,last)
      |     fprintf('%s -- Copyright %s Nexteer',NxtrConf,first)
      | else
      |     fprintf('%s -- %s%s- %s Nexteer',NxtrConf,char(169),first,last)
      | end
  Count per uSec : Constant  Value=0.01
  Data Store Read1 : DataStoreRead  DataStoreName=SimnTi
  Data Type Conversion1 : DataTypeConversion  OutDataTypeStr=uint32
  Divide1 : Product  Inputs=**
  Divide2 : Product  Inputs=*/
  Max Counts : Constant  Value=2^32-1
  Product1 : Product
  Product2 : Product
  Rounding : Rounding
  Subtract1 : Sum  Inputs=+-
  uSec per Sec : Constant  Value=1000000
  RefTmr : Outport
  wires:
  Product2/1 -> Subtract1/2
  Subtract1/1 -> Data Type Conversion1/1
  Rounding/1 -> Product2/1
  Divide2/1 -> Rounding/1
  Max Counts/1 -> Divide2/2, Product2/2
  Divide1/1 -> Divide2/1, Subtract1/1
  Product1/1 -> Divide1/1
  Count per uSec/1 -> Divide1/2
  uSec per Sec/1 -> Product1/2
  Data Type Conversion1/1 -> RefTmr/1
  Data Store Read1/1 -> Product1/1

== system SF042A_HwAgSnsrls/HwAgSnsrls/HwAgSnsrlsPer1/WhlSpdAutoCentr/WhlSpd/If Action Subsystem1/If Action Subsystem3/CopyRight2 ==

== system SF042A_HwAgSnsrls/HwAgSnsrls/HwAgSnsrlsPer1/WhlSpdAutoCentr/WhlSpd/VehSpdChk/GetTiSpan /CopyRight2 ==

== system SF042A_HwAgSnsrls/HwAgSnsrls/HwAgSnsrlsPer1/WhlSpdAutoCentr/WhlSpd/VehSpdChk/GetTiSpan /GetTiSpan100MicroSec32bit ==
  note: Subtract original reference time
  note: seconds
  note: microseconds
  note: counts
  note: Wrap-to-zero
  note: 1 count = 100 uSec
  note: Get current system time
  note: GetTiSpan100MicroSec32bit
  note: Created Aug 18, 2015
      | Modified Oct 21, 2015
      | Modified Oct 30, 2015
      | Kevin Derry
  RefTmr : Inport
  CopyRight2 : Subsystem  Description=|  mask(Copyright Information){none=on}
      | Copyright info block.                                               
      |                                                                     
      | Place copyright information at the top of every subsystem in design.
      mask prompts: none "No parameters"
      mask help: Place copyright information at the top of every subsystem in design.
      mask Display:
      | NxtrConf = 'Nexteer Confidential';
      | 
      | sys = bdroot; %handle for the current model ("system")
      | first = get_param(sys,'Created');
      | if(isempty(first))
      |     first = datestr(now,'yyyy');
      | else
      |     first = first(end-3:end);  %year is last four digits
      | end
      | 
      | last = get_param(sys,'LastModifiedDate');
      | if isempty(last)
      |     last = datestr(now,'yyyy');
      | else
      |     last = last(end-3:end);
      | end
      | 
      | if strcmp(first,last)
      |     fprintf('%s -- Copyright %s Nexteer',NxtrConf,first)
      | else
      |     fprintf('%s -- %s%s- %s Nexteer',NxtrConf,char(169),first,last)
      | end
  Count per uSec : Constant  Value=0.01
  Data Store Read1 : DataStoreRead  DataStoreName=SimnTi
  Data Type Conversion2 : DataTypeConversion  OutDataTypeStr=uint32
  Divide1 : Product  Inputs=**
  Divide2 : Product  Inputs=*/
  If : If  NumInputs=2  IfExpression=u1 >= u2
  Max Counts : Constant  Value=2^32-1
  Merge : Merge
  No wrapping : Subsystem  TreatAsAtomicUnit=on
  Product2 : Product
  Product3 : Product
  Rounding : Rounding
  Subtract3 : Sum  Inputs=+-
  Wrapping : Subsystem  TreatAsAtomicUnit=on
  uSec per Sec : Constant  Value=1000000
  TiSpan : Outport
  wires:
  Wrapping/1(Out1) -> Merge/2
  No wrapping/1(Out1) -> Merge/1
  If/2 -> Wrapping/Action
  If/1 -> No wrapping/Action
  Product3/1 -> Subtract3/2
  Subtract3/1 -> Data Type Conversion2/1
  Rounding/1 -> Product3/1
  Divide2/1 -> Rounding/1
  Max Counts/1 -> Divide2/2, Product3/2
  Divide1/1 -> Divide2/1, Subtract3/1
  Product2/1 -> Divide1/1
  Data Store Read1/1 -> Product2/1
  Count per uSec/1 -> Divide1/2
  uSec per Sec/1 -> Product2/2
  Merge/1 -> TiSpan/1
  RefTmr/1 -> If/2, No wrapping/2(ref), Wrapping/2(ref)
  Data Type Conversion2/1 -> If/1, No wrapping/1(new), Wrapping/1(new)

== system SF042A_HwAgSnsrls/HwAgSnsrls/HwAgSnsrlsPer1/WhlSpdAutoCentr/WhlSpd/VehSpdChk/Set to 0/CopyRight2 ==

== system SF042A_HwAgSnsrls/HwAgSnsrls/HwAgSnsrlsPer1/WhlSpdAutoCentr/WhlSpd/VehSpdChk/Set to 0/GetRefTmr100MicroSec32bit ==
  note: 1 count = 100 uSec
  note: seconds
  note: microseconds
  note: counts
  note: Wrap-to-zero
  note: GetRefTmr100MicroSec32bit
  note: Created Aug 18, 2015
      | Modified Oct 21, 2015
      | Modified Oct 30, 2015
      | Kevin Derry
  CopyRight2 : Subsystem  Description=|  mask(Copyright Information){none=on}
      | Copyright info block.                                               
      |                                                                     
      | Place copyright information at the top of every subsystem in design.
      mask prompts: none "No parameters"
      mask help: Place copyright information at the top of every subsystem in design.
      mask Display:
      | NxtrConf = 'Nexteer Confidential';
      | 
      | sys = bdroot; %handle for the current model ("system")
      | first = get_param(sys,'Created');
      | if(isempty(first))
      |     first = datestr(now,'yyyy');
      | else
      |     first = first(end-3:end);  %year is last four digits
      | end
      | 
      | last = get_param(sys,'LastModifiedDate');
      | if isempty(last)
      |     last = datestr(now,'yyyy');
      | else
      |     last = last(end-3:end);
      | end
      | 
      | if strcmp(first,last)
      |     fprintf('%s -- Copyright %s Nexteer',NxtrConf,first)
      | else
      |     fprintf('%s -- %s%s- %s Nexteer',NxtrConf,char(169),first,last)
      | end
  Count per uSec : Constant  Value=0.01
  Data Store Read1 : DataStoreRead  DataStoreName=SimnTi
  Data Type Conversion1 : DataTypeConversion  OutDataTypeStr=uint32
  Divide1 : Product  Inputs=**
  Divide2 : Product  Inputs=*/
  Max Counts : Constant  Value=2^32-1
  Product1 : Product
  Product2 : Product
  Rounding : Rounding
  Subtract1 : Sum  Inputs=+-
  uSec per Sec : Constant  Value=1000000
  RefTmr : Outport
  wires:
  Product2/1 -> Subtract1/2
  Subtract1/1 -> Data Type Conversion1/1
  Rounding/1 -> Product2/1
  Divide2/1 -> Rounding/1
  Max Counts/1 -> Divide2/2, Product2/2
  Divide1/1 -> Divide2/1, Subtract1/1
  Product1/1 -> Divide1/1
  Count per uSec/1 -> Divide1/2
  uSec per Sec/1 -> Product1/2
  Data Type Conversion1/1 -> RefTmr/1
  Data Store Read1/1 -> Product1/1

== system SF042A_HwAgSnsrls/HwAgSnsrls/HwAgSnsrlsPer1/VehDynAutoCentr/LpFilOneEna/VehDynTmr1/GetTiSpan1/GetTiSpan100MicroSec32bit/CopyRight2 ==

== system SF042A_HwAgSnsrls/HwAgSnsrls/HwAgSnsrlsPer1/VehDynAutoCentr/LpFilOneEna/VehDynTmr1/GetTiSpan1/GetTiSpan100MicroSec32bit/No wrapping ==
  new : Inport
  ref : Inport  Port=2
  Action Port : ActionPort  ActionType=then
  CopyRight2 : Subsystem  Description=|  mask(Copyright Information){none=on}
      | Copyright info block.                                               
      |                                                                     
      | Place copyright information at the top of every subsystem in design.
      mask prompts: none "No parameters"
      mask help: Place copyright information at the top of every subsystem in design.
      mask Display:
      | NxtrConf = 'Nexteer Confidential';
      | 
      | sys = bdroot; %handle for the current model ("system")
      | first = get_param(sys,'Created');
      | if(isempty(first))
      |     first = datestr(now,'yyyy');
      | else
      |     first = first(end-3:end);  %year is last four digits
      | end
      | 
      | last = get_param(sys,'LastModifiedDate');
      | if isempty(last)
      |     last = datestr(now,'yyyy');
      | else
      |     last = last(end-3:end);
      | end
      | 
      | if strcmp(first,last)
      |     fprintf('%s -- Copyright %s Nexteer',NxtrConf,first)
      | else
      |     fprintf('%s -- %s%s- %s Nexteer',NxtrConf,char(169),first,last)
      | end
  Subtract1 : Sum  Inputs=+-
  Out1 : Outport
  wires:
  ref/1 -> Subtract1/2
  new/1 -> Subtract1/1
  Subtract1/1 -> Out1/1

== system SF042A_HwAgSnsrls/HwAgSnsrls/HwAgSnsrlsPer1/VehDynAutoCentr/LpFilOneEna/VehDynTmr1/GetTiSpan1/GetTiSpan100MicroSec32bit/Wrapping ==
  new : Inport
  ref : Inport  Port=2
  Action Port : ActionPort  ActionType=else
  CopyRight2 : Subsystem  Description=|  mask(Copyright Information){none=on}
      | Copyright info block.                                               
      |                                                                     
      | Place copyright information at the top of every subsystem in design.
      mask prompts: none "No parameters"
      mask help: Place copyright information at the top of every subsystem in design.
      mask Display:
      | NxtrConf = 'Nexteer Confidential';
      | 
      | sys = bdroot; %handle for the current model ("system")
      | first = get_param(sys,'Created');
      | if(isempty(first))
      |     first = datestr(now,'yyyy');
      | else
      |     first = first(end-3:end);  %year is last four digits
      | end
      | 
      | last = get_param(sys,'LastModifiedDate');
      | if isempty(last)
      |     last = datestr(now,'yyyy');
      | else
      |     last = last(end-3:end);
      | end
      | 
      | if strcmp(first,last)
      |     fprintf('%s -- Copyright %s Nexteer',NxtrConf,first)
      | else
      |     fprintf('%s -- %s%s- %s Nexteer',NxtrConf,char(169),first,last)
      | end
  Max Counts : Constant  Value=2^32-1  OutDataTypeStr=uint32
  Subtract1 : Sum  Inputs=+-+
  Out1 : Outport
  wires:
  new/1 -> Subtract1/3
  ref/1 -> Subtract1/2
  Max Counts/1 -> Subtract1/1
  Subtract1/1 -> Out1/1

== system SF042A_HwAgSnsrls/HwAgSnsrls/HwAgSnsrlsPer1/VehDynAutoCentr/LpFilOneEna/VehDynTmr1/If Action Subsystem3/GetRefTmr100MicroSec32bit/CopyRight2 ==

== system SF042A_HwAgSnsrls/HwAgSnsrls/HwAgSnsrlsPer1/VehDynAutoCentr/LpFilOneEna/VehDynTmr1/Set to 0/GetRefTmr100MicroSec32bit/CopyRight2 ==

== system SF042A_HwAgSnsrls/HwAgSnsrls/HwAgSnsrlsPer1/VehDynAutoCentr/LpFilTwoEna/VehDynTmr2/GetTiSpan2/GetTiSpan100MicroSec32bit/CopyRight2 ==
